simulink library "groundStation000_cl"  (R2018b)
settings: Solver=VariableStepAuto  StartTime=0.0  StopTime=10.0  RelTol=1e-3
undefined symbols (not defined in the file): thr
libraries: eulAng2RotMat_ul x1, massSpringDamper_ul x1, tethersMoment_cl x1, nodePosToLinkPos_ul x1, thrAttachPtKinematics_ul x1
settings Model: Creator=M.Cobb  LastModifiedBy=jcreed2

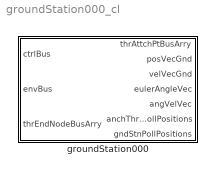
== system groundStation000_cl ==
  groundStation000 : Subsystem  mask{gs=0}
      mask prompts: gs "Ground station object"

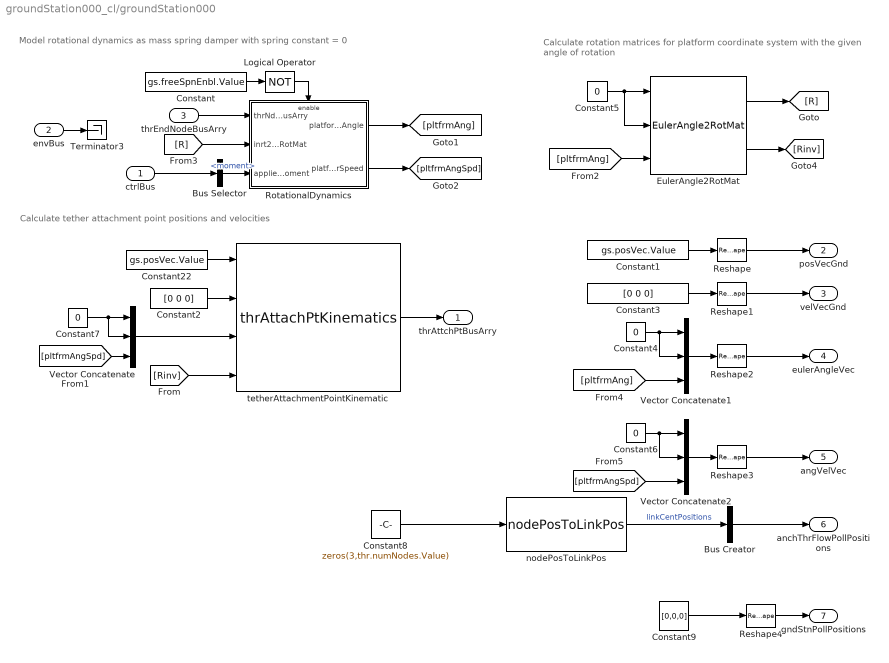
== system groundStation000_cl/groundStation000 ==
  note: Calculate tether attachment point positions and velocities
  note: Calculate rotation matrices for platform coordinate
      | system with the given angle of rotation
  note: Model rotational dynamics as mass spring damper with
      | spring constant = 0
  ctrlBus : Inport  OutDataTypeStr=Bus: gndStnCtrlBus
  envBus : Inport  Port=2  OutDataTypeStr=Bus: envBus
  thrEndNodeBusArry : Inport  Port=3
  Bus Creator : BusCreator  Inputs=1  OutDataTypeStr=Bus: thrPollPosBus  NonVirtualBus=on
  Bus Selector : BusSelector  OutputSignals=moment
  Constant : Constant  Value=gs.freeSpnEnbl.Value
  Constant1 : Constant  Value=gs.posVec.Value
  Constant2 : Constant  Value=[0 0 0]
  Constant22 : Constant  Value=gs.posVec.Value
  Constant3 : Constant  Value=[0 0 0]
  Constant{4..7} (4 alike) : Constant  Value=0
  Constant8 : Constant  Value=zeros(3,thr.numNodes.Value)
  Constant9 : Constant  Value=[0,0,0]
  EulerAngle2RotMat : eulAng2RotMat_ul/EulerAngle2RotMat  SystemSampleTime=-1
  Logical Operator : Logic  Operator=NOT  AllPortsSameDT=off  OutDataTypeStr=boolean
  Reshape{,1..4} (5 alike) : Reshape  OutputDimensionality=Column vector (2-D)
  RotationalDynamics : Subsystem
      settings: MinAlgLoopOccurrences=on
  Terminator3 : Terminator
  Vector Concatenate : Concatenate  NumInputs=3
  Vector Concatenate1 : Concatenate  NumInputs=3
  Vector Concatenate2 : Concatenate  NumInputs=3
  nodePosToLinkPos : nodePosToLinkPos_ul/nodePosToLinkPos  SystemSampleTime=-1
  tetherAttachmentPointKinematic : thrAttachPtKinematics_ul/thrAttachPtKinematics  atchPts=gs.struct('OCT.thrAttch')
  thrAttchPtBusArry : Outport
  posVecGnd : Outport  Port=2
  velVecGnd : Outport  Port=3
  eulerAngleVec : Outport  Port=4
  angVelVec : Outport  Port=5
  anchThrFlowPollPositions : Outport  Port=6
  gndStnPollPositions : Outport  Port=7
  wires:
  Constant5/1 -> EulerAngle2RotMat/2, EulerAngle2RotMat/1
  EulerAngle2RotMat/1 -> [R]
  EulerAngle2RotMat/2 -> [Rinv]
  Constant7/1 -> Vector Concatenate/1, Vector Concatenate/2
  tetherAttachmentPointKinematic/1 -> thrAttchPtBusArry/1
  Constant22/1 -> tetherAttachmentPointKinematic/1
  Constant2/1 -> tetherAttachmentPointKinematic/2
  [Rinv] -> tetherAttachmentPointKinematic/4
  Vector Concatenate/1 -> tetherAttachmentPointKinematic/3
  [pltfrmAngSpd] -> Vector Concatenate/3
  [pltfrmAng] -> EulerAngle2RotMat/3
  ctrlBus/1 -> Bus Selector/1
  envBus/1 -> Terminator3/1
  Constant/1 -> Logical Operator/1
  Logical Operator/1 -> RotationalDynamics/Enable
  thrEndNodeBusArry/1 -> RotationalDynamics/1(thrNdFrcBusArry)
  [R] -> RotationalDynamics/2(inrt2BdyRotMat)
  RotationalDynamics/1(platformAngle) -> [pltfrmAng]
  RotationalDynamics/2(platformAngularSpeed) -> [pltfrmAngSpd]
  Constant1/1 -> Reshape/1
  Reshape/1 -> posVecGnd/1
  Reshape1/1 -> velVecGnd/1
  Reshape2/1 -> eulerAngleVec/1
  Reshape3/1 -> angVelVec/1
  Constant3/1 -> Reshape1/1
  Vector Concatenate1/1 -> Reshape2/1
  Constant4/1 -> Vector Concatenate1/2, Vector Concatenate1/1
  Constant6/1 -> Vector Concatenate2/1, Vector Concatenate2/2
  Vector Concatenate2/1 -> Reshape3/1
  [pltfrmAng] -> Vector Concatenate1/3
  [pltfrmAngSpd] -> Vector Concatenate2/3
  Bus Selector/1 -> RotationalDynamics/3(appliedMoment)  "<moment>"
  Bus Creator/1 -> anchThrFlowPollPositions/1
  nodePosToLinkPos/1 -> Bus Creator/1  "linkCentPositions"
  Constant8/1 -> nodePosToLinkPos/1
  Constant9/1 -> Reshape4/1
  Reshape4/1 -> gndStnPollPositions/1

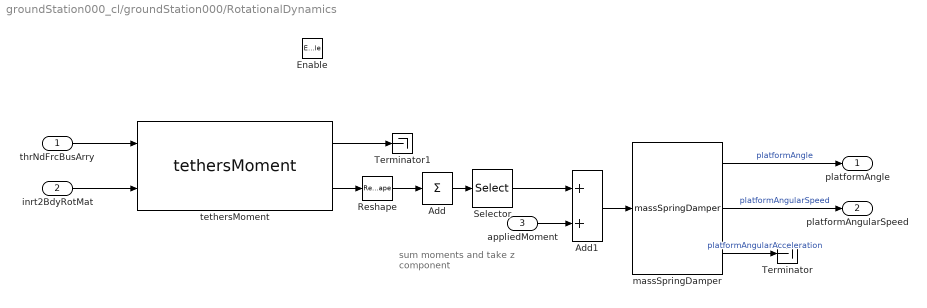
== system groundStation000_cl/groundStation000/RotationalDynamics ==
  note: sum moments and
      | take z component
  thrNdFrcBusArry : Inport
  inrt2BdyRotMat : Inport  Port=2
  appliedMoment : Inport  Port=3
  Enable : EnablePort
  Add : Sum  Inputs=+  CollapseMode=Specified dimension  CollapseDim=2
  Add1 : Sum
  Reshape : Reshape  OutputDimensionality=Customize  OutputDimensions=[3 gs.numTethers.Value]
  Selector : Selector  InputPortWidth=3  IndexOptions=Index vector (dialog)  Indices=3  OutputSizes=1
  Terminator : Terminator
  Terminator1 : Terminator
  massSpringDamper : massSpringDamper_ul/massSpringDamper  m=gs.inertia.Value  b=gs.dampCoeff.Value  k=0  x0=gndStn.initAngPos.Value  xDot0=gndStn.initAngPos.Value
  tethersMoment : tethersMoment_cl/tethersMoment  arms=gs.struct('OCT.thrAttch')
  platformAngle : Outport  InitialOutput=gs.initAngPos.Value
  platformAngularSpeed : Outport  Port=2  InitialOutput=gs.initAngVel.Value
  wires:
  massSpringDamper/2 -> platformAngularSpeed/1  "platformAngularSpeed"
  Add/1 -> Selector/1
  Selector/1 -> Add1/1
  Reshape/1 -> Add/1
  tethersMoment/1 -> Terminator1/1
  tethersMoment/2 -> Reshape/1
  thrNdFrcBusArry/1 -> tethersMoment/1
  inrt2BdyRotMat/1 -> tethersMoment/2
  massSpringDamper/1 -> platformAngle/1  "platformAngle"
  massSpringDamper/3 -> Terminator/1  "platformAngularAcceleration"
  Add1/1 -> massSpringDamper/1
  appliedMoment/1 -> Add1/2
